simulink model "ibrir"  (R2024b)
settings: Solver=VariableStepAuto  StartTime=0.0  StopTime=10.0  RelTol=1e-3
libraries: simulink x1
settings Model: Creator=user  LastModifiedBy=user

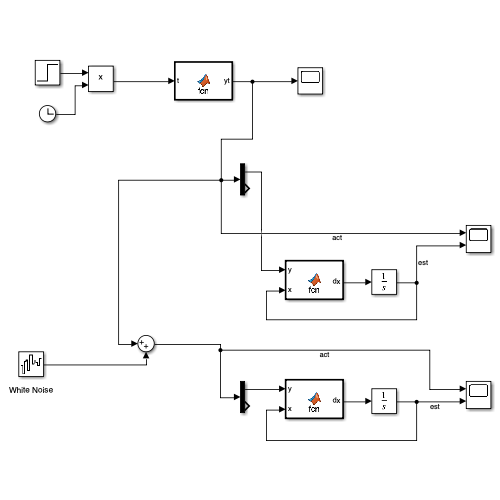
[thumbnail: Simulink's stored preview of the top-level diagram]
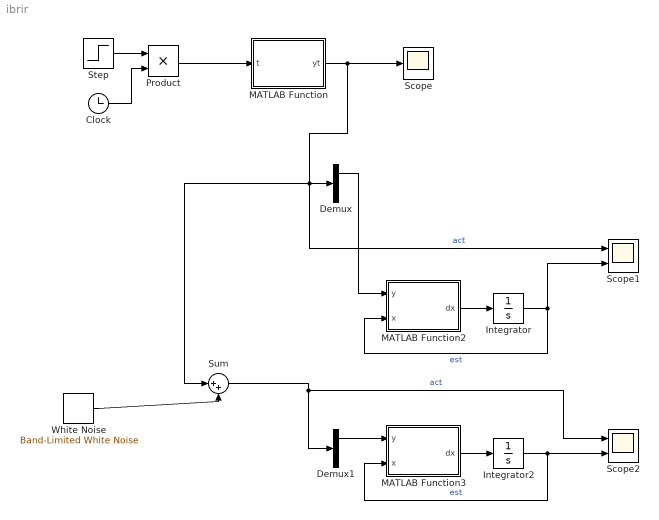
== system ibrir ==
  " White Noise" : simulink/Sources/Band-Limited White Noise  Cov=[0.1]  Ts=0.001  seed=[23341]
  Clock : Clock
  Demux : Demux  Outputs=[1, 3]
  Demux1 : Demux  Outputs=[1, 3]
  Integrator : Integrator
  Integrator2 : Integrator
  MATLAB Function : MATLAB Function  TreatAsAtomicUnit=on
  MATLAB Function2 : MATLAB Function  TreatAsAtomicUnit=on
  MATLAB Function3 : MATLAB Function  TreatAsAtomicUnit=on
  Product : Product
  Scope : Scope
  Scope1 : Scope  NumInputPorts=2
  Scope2 : Scope  NumInputPorts=2
  Step : Step  Time=0  SampleTime=0.001
  Sum : Sum  Inputs=|++
  wires:
  MATLAB Function/1(yt) -> Scope1/1, Sum/1, Demux/1, Scope/1  "act"
  Step/1 -> Product/1
  Product/1 -> MATLAB Function/1(t)
  Clock/1 -> Product/2
  Demux/1 -> MATLAB Function2/1(y)
  MATLAB Function2/1(dx) -> Integrator/1
  Integrator/1 -> MATLAB Function2/2(x), Scope1/2  "est"
  " White Noise"/1 -> Sum/2
  Sum/1 -> Scope2/1, Demux1/1  "act"
  MATLAB Function3/1(dx) -> Integrator2/1
  Integrator2/1 -> Scope2/2, MATLAB Function3/2(x)  "est"
  Demux1/1 -> MATLAB Function3/1(y)

== matlab function ibrir/MATLAB Function2 ==
  data: y input; dx output; x input
function dx = fcn(y, x)
    % Parameters
    n = 4;                % Order of the observer
    epsilon = 1/200;      % Small gain parameter
    k = [4, 6, 4, 1];     % Binomial coefficients (for n = 4)

    % Initialize output derivative
    dx = zeros(n, 1);
    
    % High-Gain Observer Equations
    dx(1) = x(2) + (k(1) / epsilon^1) * (y - x(1));
    dx(2) = x(3) + (k(2) / epsilon^2) * (y - x(1));
    dx(3) = x(4) + (k(3) / epsilon^3) * (y - x(1));
    dx(4) = (k(4) / epsilon^4) * (y - x(1));
end

== matlab function ibrir/MATLAB Function3 ==
  data: y input; dx output; x input
function dx = fcn(y, x)
    % Parameters
    n = 4;                % Order of the observer
    epsilon = 1/20;      % Small gain parameter
    k = [4, 6, 4, 1];     % Binomial coefficients (for n = 4)

    % Initialize output derivative
    dx = zeros(n, 1);
    
    % High-Gain Observer Equations
    dx(1) = x(2) + (k(1) / epsilon^1) * (y - x(1));
    dx(2) = x(3) + (k(2) / epsilon^2) * (y - x(1));
    dx(3) = x(4) + (k(3) / epsilon^3) * (y - x(1));
    dx(4) = (k(4) / epsilon^4) * (y - x(1));
end

== matlab function ibrir/MATLAB Function ==
  data: t input; yt output
function yt = fcn(t)

y = sin(t) + cos(5*t);
dy = cos(t) - 5*sin(5*t);
d2y = -sin(t) - 25*cos(5*t);
d3y = -cos(t) + 125*sin(5*t);
%d4y = sin(t) + 625*cos(5*t);

yt = [y; dy; d2y; d3y];
